simulink model "PredatorPreyModel_SIM"  (R2012b)
settings: Solver=ode3  StartTime=0.0  StopTime=10.0  FixedStep=0.1  RelTol=1e-3
values from neighbouring files (symbols this model uses):
  predator0 = ic(2, i)    [PredatorPreyModel.m]
  prey0 = ic(1, i)    [PredatorPreyModel.m]
settings Model: Creator=aluno  LastModifiedBy=aluno

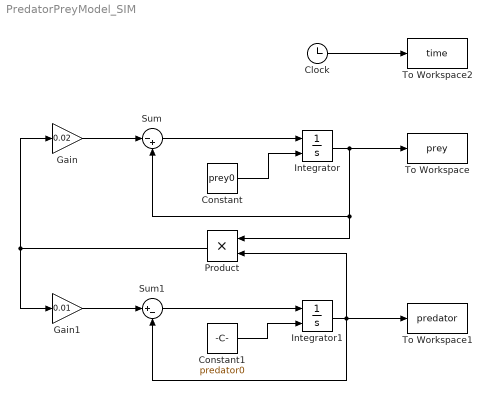
== system PredatorPreyModel_SIM ==
  Clock : Clock
  Constant : Constant  Value=prey0
  Constant1 : Constant  Value=predator0
  Gain : Gain  Gain=0.02
  Gain1 : Gain  Gain=0.01
  Integrator : Integrator  InitialConditionSource=external
  Integrator1 : Integrator  InitialConditionSource=external
  Product : Product  RndMeth=Zero
  Sum : Sum  Inputs=|-+
  Sum1 : Sum  Inputs=|+-
  To Workspace : ToWorkspace  VariableName=prey  SampleTime=-1
  To Workspace1 : ToWorkspace  VariableName=predator  SampleTime=-1
  To Workspace2 : ToWorkspace  VariableName=time  SampleTime=-1
  wires:
  Constant/1 -> Integrator/2
  Sum1/1 -> Integrator1/1
  Constant1/1 -> Integrator1/2
  Gain1/1 -> Sum1/1
  Product/1 -> Gain/1, Gain1/1
  Gain/1 -> Sum/1
  Sum/1 -> Integrator/1
  Integrator/1 -> To Workspace/1, Sum/2, Product/1
  Integrator1/1 -> To Workspace1/1, Sum1/2, Product/2
  Clock/1 -> To Workspace2/1
